simulink model "FCS_Sim"  (R2024a)
settings: Solver=FixedStepAuto  StartTime=0.0  StopTime=30  FixedStep=Sim.samp_T  MaxStep=1e-2  RelTol=1e-3  AbsTol=1e-3
StopFcn:
  | combineMatFiles(Sim.output_name)
libraries: simulink x1
settings Model: Creator=gurt1  LastModifiedBy=gurt1
settings OptimizationCC: DefaultParameterBehavior=Inlined  EnhancedBackFolding=on  PassReuseOutputArgsAs=Individual arguments  ZeroExternalMemoryAtStartup=off  ZeroInternalMemoryAtStartup=off  MaxStackSize=64  OptimizeBlockOrder=speed  DifferentSizesBufferReuse=on  OptimizationCustomize=off  EfficientTunableParamExpr=on
settings DebuggingCC: ParameterTunabilityLossMsg=error
settings HardwareCC: ProdBitPerPointer=32  ProdBitPerSizeT=32  ProdBitPerPtrDiffT=32  ProdLargestAtomicInteger=Long  ProdLargestAtomicFloat=Double  ProdWordSize=32  ProdHWDeviceType=ARM Compatible->ARM Cortex
settings RTWCC: Description=Embedded Coder  SystemTargetFile=ert.tlc  TemplateMakefile=ert_default_tmf  Toolchain=GNU Tools for PX4 Autopilots  GPUComputeCapability=3.5
settings CodeAppCC: ForceParamTrailComments=on  IgnoreCustomStorageClasses=off  OperatorAnnotations=on  SimulinkDataObjDesc=on  SFDataObjDesc=on  InsertBlockDesc=on
settings ERTTargetCC: ExtModeTransport=3  ExtModeStaticAlloc=on  ExtModeMexFile=ext_xcp  ExtModeIntrfLevel=Level2 - Open  ERTCustomFileTemplate=example_file_process.tlc

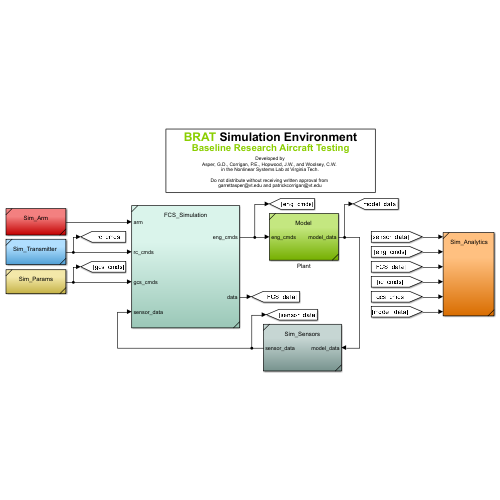
[thumbnail: Simulink's stored preview of the top-level diagram]
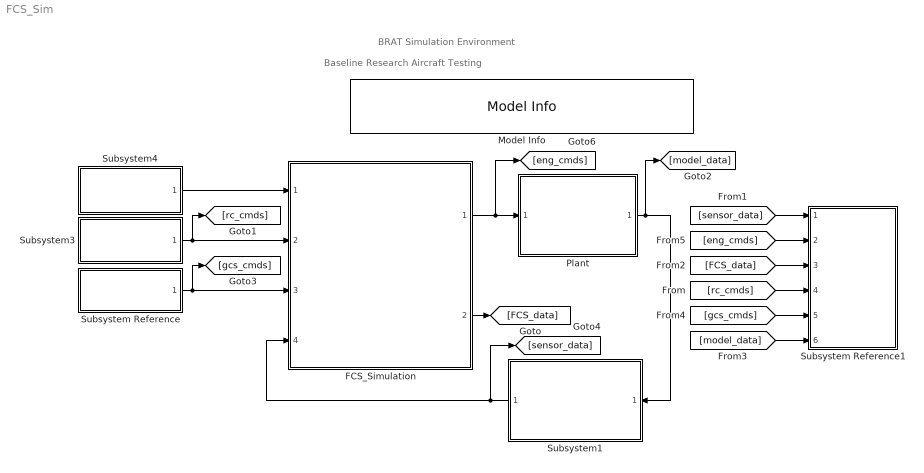
== system FCS_Sim ==
  note: BRAT Simulation Environment
  note: Baseline Research Aircraft Testing
  FCS_Simulation : Subsystem  ReferencedSubsystem=FCS_Simulation
  Model Info : simulink/Model-Wide Utilities/Model Info  Frame=off  DisplayStringWithTags=|  HorizontalTextAlignment=Center  LeftAlignmentValue=0.5
      | Developed by
      | Asper, G.D., Corrigan, P.E., Hopwood, J.W., and Woolsey, C.W. 
      | in the Nonlinear Systems Lab at Virginia Tech.
      | 
      | Do not distribute without receiving written approval from 
      | garrettasper@vt.edu and patrickcorrigan@vt.edu
  Plant : Subsystem  ReferencedSubsystem=Model
  Subsystem Reference : Subsystem  ReferencedSubsystem=Sim_Params
  Subsystem Reference1 : Subsystem  ReferencedSubsystem=Sim_Analytics
  Subsystem1 : Subsystem  ReferencedSubsystem=Sim_Sensors
  Subsystem3 : Subsystem  ReferencedSubsystem=Sim_Transmitter
  Subsystem4 : Subsystem  ReferencedSubsystem=Sim_Arm
  wires:
  Subsystem4/1 -> FCS_Simulation/1
  Subsystem3/1 -> [rc_cmds], FCS_Simulation/2
  Subsystem1/1 -> FCS_Simulation/4, [sensor_data]
  Subsystem Reference/1 -> [gcs_cmds], FCS_Simulation/3
  FCS_Simulation/1 -> [eng_cmds], Plant/1
  FCS_Simulation/2 -> [FCS_data]
  Plant/1 -> [model_data], Subsystem1/1
  [sensor_data] -> Subsystem Reference1/1
  [eng_cmds] -> Subsystem Reference1/2
  [FCS_data] -> Subsystem Reference1/3
  [rc_cmds] -> Subsystem Reference1/4
  [gcs_cmds] -> Subsystem Reference1/5
  [model_data] -> Subsystem Reference1/6
